simulink model "nb_spect_r2"  (R2012b)
settings: Solver=ode45  StartTime=0.0  StopTime=50000  RelTol=1e-3
undefined symbols (not defined in the file): pfb_coeff_gen_calc, sigbuilder_block, xlipgetpartsetting
libraries: xbsIndex_r4 x12159, casper_library_misc x81, casper_library_delays x40, simulink x17, dspsigops x12, xps_library x8, xbsReplacements_r4 x4, casper_library_flow_control x2
(part 6 of 142)

== system nb_spect_r2/packetizer ==
  din_valid : Inport
  din : Inport  Port=2
  reset : Inport  Port=3
  Counter : xbsIndex_r4/Counter  cnt_type=Free Running  cnt_to=Inf  operation=Up  start_count=0  cnt_by_val=1  arith_type=Unsigned  n_bits=11  bin_pt=0  load_pin=off  rst=on  en=on  explicit_period=on  period=1  dbl_ovrd=off  use_behavioral_HDL=off  implementation=Fabric  use_rpm=off  block_type=counter
  Inverter : xbsIndex_r4/Inverter  en=off  latency=0  dbl_ovrd=off  block_type=inv
  Logical : xbsIndex_r4/Logical  logical_function=AND  inputs=2  en=off  latency=0  precision=Full  arith_type=Unsigned  n_bits=16  bin_pt=0  align_bp=on  dbl_ovrd=off  block_type=logical
  Logical1 : xbsIndex_r4/Logical  logical_function=AND  inputs=2  en=off  latency=0  precision=Full  arith_type=Unsigned  n_bits=16  bin_pt=0  align_bp=on  dbl_ovrd=off  block_type=logical
  control_fsm : xbsIndex_r4/MCode  mfname=packetizer_fsm  explicit_period=on  period=1  inputsTable={'boundInpExpr'=>['','','3','',' 2047 ',''],'inputs'=>['fifo_empty','shift_count','data_per_word','data_count','n_words','reset']}  outputsTable={'outputs'=>['fifo_re','bram_addr_en','bram_we','serializer_shift','serializer_ld','shift_count_en','shift_count_rst','bram_addr_rst','data_count_en','data_count_rst','done'],'suppressOut'=>['off','off','off','off','off','off','off','off','off','off','off']}  dbl_ovrd=off  enable_stdout=off  enable_debug=off  suppress_output=1  defparams={'data_per_word',1, 'n_words', 8191 }  hide_port_list={}  block_type=mcode
      settings: block_version=10.1.3
  data_buffer : xbsIndex_r4/FIFO  mem_type=Block RAM  performance_options=Standard_FIFO  infoedit1=Available only for V4, V5, V6, V7, K7, A7 and Zynq devices.  embedded_registers=off  depth=4K  percent_nbits=8  rst=on  en=off  use_dcount=off  use_percent_full_port=on  use_almost_empty=off  almost_empty_thresh=2  use_almost_full=off  almost_full_thresh=14  dbl_ovrd=off  explicit_period=off  block_type=fifo
      settings: block_version=10.1.3
  data_counter : xbsIndex_r4/Counter  cnt_type=Free Running  cnt_to=Inf  operation=Up  start_count=0  cnt_by_val=1  arith_type=Unsigned  n_bits=14  bin_pt=0  load_pin=off  rst=on  en=on  explicit_period=on  period=1  dbl_ovrd=off  use_behavioral_HDL=off  implementation=Fabric  use_rpm=off  block_type=counter
  parallel_to_serial_converter : Subsystem  AncestorBlock=casper_library_flow_control/parallel_to_serial_converter  mask(parallel_to_serial_converter){pin_width=128, sout_width=64}
      mask prompts: pin_width "Parallel Input Width"; sout_width "Serial Output Width"
      mask help:
      | This block takes as input a parallel bus of specified width.
      | When the load signal 'ld' is asserted, this data is broken into
      | pieces of width specified by the serial output width and
      | stored into different registers chained to form a shift register.
      | If the 'shift' input is subsequently asserted, the shift register
      | returns as output a new piece of data of width sout_width.  This data
      | is the next least significant piece of the original bus.  The converter
      | serializes SMALL ENDIAN.
      |
      | Note that the load operation automatically loads the least significant
      | bits into the register closest to the output, so the first 'shift'
      | assertion changes the data output from bits [sout_width-1:0] to
      | bits [2*sout_width-1:sout_width].
      mask init:
      | parallel_to_serial_converter_init(gcb, ...
      |     'pin_width', pin_width, ...
      |     'sout_width', sout_width);
  shift_counter : xbsIndex_r4/Counter  cnt_type=Free Running  cnt_to=Inf  operation=Up  start_count=0  cnt_by_val=1  arith_type=Unsigned  n_bits=1  bin_pt=0  load_pin=off  rst=on  en=on  explicit_period=on  period=1  dbl_ovrd=off  use_behavioral_HDL=off  implementation=Fabric  use_rpm=off  block_type=counter
  data_addr : Outport
  data_sout : Outport  Port=2
  data_valid : Outport  Port=3
  buffer_overflow : Outport  Port=4
  perc_full : Outport  Port=5
  done : Outport  Port=6
  wires:
  control_fsm/10 -> data_counter/1
  reset/1 -> data_buffer/4, control_fsm/4
  data_counter/1 -> control_fsm/3
  control_fsm/9 -> data_counter/2
  control_fsm/8 -> Counter/1
  control_fsm/2 -> Counter/2
  Counter/1 -> data_addr/1
  data_buffer/2 -> control_fsm/1
  control_fsm/7 -> shift_counter/1
  shift_counter/1 -> control_fsm/2
  control_fsm/6 -> shift_counter/2
  parallel_to_serial_converter/1(sout) -> data_sout/1
  din/1 -> data_buffer/1
  control_fsm/3 -> data_valid/1
  control_fsm/5 -> parallel_to_serial_converter/2(ld)
  control_fsm/4 -> parallel_to_serial_converter/3(shift)
  control_fsm/1 -> data_buffer/3
  data_buffer/1 -> parallel_to_serial_converter/1(pin)
  Logical/1 -> data_buffer/2
  din_valid/1 -> Logical/1, Logical1/1
  Inverter/1 -> Logical/2
  data_buffer/4 -> Inverter/1, Logical1/2
  Logical1/1 -> buffer_overflow/1
  data_buffer/3 -> perc_full/1
  control_fsm/11 -> done/1

== system nb_spect_r2/pfb_fir_async ==
  sync : Inport
  dv : Inport  Port=2
  pol1_in1 : Inport  Port=3
  dv_delay : xbsIndex_r4/Delay  rst=off  infoeditControl=Selection of Reset will increase slice count due to use of real FFs and instead of SRLs  en=off  latency=bram_latency+1  dbl_ovrd=off  reg_retiming=off  block_type=delay
      settings: block_version=11.4
  pol1_in1_coeffs : Subsystem  AncestorBlock=casper_library_pfbs/pfb_coeff_gen  mask(pfb_coeff_gen){PFBSize=12, CoeffBitWidth=8, TotalTaps=6, CoeffDistMem=off, WindowType=hann, bram_latency=3, n_inputs=0, nput=0, fwidth=1, debug_mode=off, fan_latency=3}
      mask prompts: PFBSize "Size of PFB: (2^? pnts)"; CoeffBitWidth "Bitwidth of Coefficients:"; TotalTaps "Total Number of Taps:"; CoeffDistMem "Implement Coeff Gen in Distributed Memory"; WindowType "Windowing Function:"; bram_latency "BRAM Latency"; n_inputs "Number of Simultaneous Inputs: (2^?)"; nput "This is input number:"; fwidth "Bin Width (normal=1)"; debug_mode "Debug mode - coeffs are a [1:pfb_size*taps] ramp."; fan_latency "Fanout latency"
      mask init:
      | pfb_coeff_gen_init(gcb, ...
      |     'PFBSize', PFBSize, ...
      |     'CoeffBitWidth', CoeffBitWidth, ...
      |     'TotalTaps', TotalTaps, ...
      |     'CoeffDistMem', CoeffDistMem, ...
      |     'WindowType', WindowType, ...
      |     'bram_latency', bram_latency, ...
      |     'n_inputs', n_inputs, ...
      |     'nput', nput, ...
      |     'fwidth', fwidth, ...
      |     'fan_latency', fan_latency, ...
      |     'debug_mode', debug_mode);
      settings: AttributesFormatString=|
      | PFBSize=12, n_inputs=0,
      | taps=6, input=0
  pol1_in1_last_tap : Subsystem  AncestorBlock=casper_library_pfbs/last_tap_async  mask(last_tap_async){input_num=1, total_taps=6, data_in_bits=18, data_out_bits=18, coeff_bits=8, add_latency=3, mult_latency=5, quantization=Round  (unbiased: Even Values), use_hdl=on, use_embedded=off, async=on, debug_mode=off}
      mask prompts: input_num "Input number:"; total_taps "Total Number of Taps:"; data_in_bits "Input Bitwidth:"; data_out_bits "Output Bitwidth:"; coeff_bits "Coeff Bitwidth:"; add_latency "Add Latency"; mult_latency "Mult Latency"; quantization "Quantization Behavior"; use_hdl "Use behavioral HDL for multlipliers"; use_embedded "Use embedded multipliers"; async "Make asynchronous?"; debug_mode "Debug mode - coeffs are a [1:pfb_size*taps] ramp."
      mask init:
      | last_tap_async_init(gcb,...
      |     'input_num', input_num, ...
      |     'total_taps', total_taps,...
      |     'data_in_bits', data_in_bits,...
      |     'data_out_bits', data_out_bits,...
      |     'coeff_bits', coeff_bits,...
      |     'add_latency', add_latency,...
      |     'mult_latency', mult_latency,...
      |     'quantization', quantization,...
      |     'use_hdl', use_hdl,...
      |     'use_embedded', use_embedded, ...
      |     'async', async, ...
      |     'debug_mode', debug_mode);
      settings: AttributesFormatString=input(1), tap(6,6)
      mask TypeOptions quantization: Truncate | Round  (unbiased: +/- Inf) | Round  (unbiased: Even Values)
      mask Callback use_hdl:
      | use_hdl = get_param(gcb,'use_hdl');
      | if( strcmp(use_hdl,'on')),
      |     set_param(gcb, 'use_embedded','off');
      |     set_param(gcb, 'MaskVisibilities',{'on','on','on','on','on','on','on','on','on','off', 'on', 'on'});
      | else
      |     set_param(gcb, 'MaskVisibilities',{'on','on','on','on','on','on','on','on','on','on', 'on', 'on'});
      | end
  pol1_in1_tap1 : Subsystem  AncestorBlock=casper_library_pfbs/tap_async  mask(tap_async){this_tap=1, pfb_bits=12, coeff_bits=8, total_taps=6, data_in_bits=18, mult_latency=5, bram_latency=3, simul_bits=0, fwidth=1, use_hdl=on, use_embedded=off, async=on, debug_mode=off}
      mask prompts: this_tap "Tap number:"; pfb_bits "Size of PFB: (2^? pnts)"; coeff_bits "Bitwidth of Coefficients:"; total_taps "Total Number of Taps:"; data_in_bits "Input Bitwidth:"; mult_latency "Mult Latency"; bram_latency "BRAM Latency"; simul_bits "Number of Simultaneous Inputs: (2^?)"; fwidth "Bit Width (normal=1)"; use_hdl "Use behavioral HDL for multlipliers"; use_embedded "Use embedded multipliers"; async "Make asynchronous?"; debug_mode "Debug mode - coeffs are a [1:pfb_size*taps] ramp."
      mask init:
      | pfb_async_tap_init(gcb,...
      |     'this_tap', this_tap, ...
      |     'pfb_bits', pfb_bits,...
      |     'coeff_bits', coeff_bits,...
      |     'total_taps', total_taps,...
      |     'data_in_bits', data_in_bits,...
      |     'mult_latency', mult_latency,...
      |     'bram_latency', bram_latency,...
      |     'simul_bits', simul_bits,...
      |     'fwidth', fwidth,...
      |     'use_hdl', use_hdl,...
      |     'use_embedded', use_embedded,...
      |     'async', async, ...
      |     'debug_mode', debug_mode);
      settings: AttributesFormatString=tap(1/6)
      mask Callback use_hdl:
      | use_hdl = get_param(gcb,'use_hdl');
      | if( strcmp(use_hdl,'on')),
      |     set_param(gcb, 'use_embedded','off');
      |     set_param(gcb, 'MaskVisibilities',{'on','on','on','on','on','on','on','on','on','on','off','on', 'on'});
      | else,
      |     set_param(gcb, 'MaskVisibilities',{'on','on','on','on','on','on','on','on','on','on','on','on', 'on'});
      | end
  pol1_in1_tap2 : Subsystem  AncestorBlock=casper_library_pfbs/tap_async  mask(tap_async){this_tap=2, pfb_bits=12, coeff_bits=8, total_taps=6, data_in_bits=18, mult_latency=5, bram_latency=3, simul_bits=0, fwidth=1, use_hdl=on, use_embedded=off, async=on, debug_mode=off}
      mask prompts: this_tap "Tap number:"; pfb_bits "Size of PFB: (2^? pnts)"; coeff_bits "Bitwidth of Coefficients:"; total_taps "Total Number of Taps:"; data_in_bits "Input Bitwidth:"; mult_latency "Mult Latency"; bram_latency "BRAM Latency"; simul_bits "Number of Simultaneous Inputs: (2^?)"; fwidth "Bit Width (normal=1)"; use_hdl "Use behavioral HDL for multlipliers"; use_embedded "Use embedded multipliers"; async "Make asynchronous?"; debug_mode "Debug mode - coeffs are a [1:pfb_size*taps] ramp."
      mask init: same as nb_spect_r2/pfb_fir_async/pol1_in1_tap1
      settings: AttributesFormatString=tap(2/6)
      mask Callback use_hdl:
      | use_hdl = get_param(gcb,'use_hdl');
      | if( strcmp(use_hdl,'on')),
      |     set_param(gcb, 'use_embedded','off');
      |     set_param(gcb, 'MaskVisibilities',{'on','on','on','on','on','on','on','on','on','on','off','on', 'on'});
      | else,
      |     set_param(gcb, 'MaskVisibilities',{'on','on','on','on','on','on','on','on','on','on','on','on', 'on'});
      | end
  pol1_in1_tap3 : Subsystem  AncestorBlock=casper_library_pfbs/tap_async  mask(tap_async){this_tap=3, pfb_bits=12, coeff_bits=8, total_taps=6, data_in_bits=18, mult_latency=5, bram_latency=3, simul_bits=0, fwidth=1, use_hdl=on, use_embedded=off, async=on, debug_mode=off}
      mask prompts: this_tap "Tap number:"; pfb_bits "Size of PFB: (2^? pnts)"; coeff_bits "Bitwidth of Coefficients:"; total_taps "Total Number of Taps:"; data_in_bits "Input Bitwidth:"; mult_latency "Mult Latency"; bram_latency "BRAM Latency"; simul_bits "Number of Simultaneous Inputs: (2^?)"; fwidth "Bit Width (normal=1)"; use_hdl "Use behavioral HDL for multlipliers"; use_embedded "Use embedded multipliers"; async "Make asynchronous?"; debug_mode "Debug mode - coeffs are a [1:pfb_size*taps] ramp."
      mask init: same as nb_spect_r2/pfb_fir_async/pol1_in1_tap1
      settings: AttributesFormatString=tap(3/6)
      mask Callback use_hdl:
      | use_hdl = get_param(gcb,'use_hdl');
      | if( strcmp(use_hdl,'on')),
      |     set_param(gcb, 'use_embedded','off');
      |     set_param(gcb, 'MaskVisibilities',{'on','on','on','on','on','on','on','on','on','on','off','on', 'on'});
      | else,
      |     set_param(gcb, 'MaskVisibilities',{'on','on','on','on','on','on','on','on','on','on','on','on', 'on'});
      | end
  pol1_in1_tap4 : Subsystem  AncestorBlock=casper_library_pfbs/tap_async  mask(tap_async){this_tap=4, pfb_bits=12, coeff_bits=8, total_taps=6, data_in_bits=18, mult_latency=5, bram_latency=3, simul_bits=0, fwidth=1, use_hdl=on, use_embedded=off, async=on, debug_mode=off}
      mask prompts: this_tap "Tap number:"; pfb_bits "Size of PFB: (2^? pnts)"; coeff_bits "Bitwidth of Coefficients:"; total_taps "Total Number of Taps:"; data_in_bits "Input Bitwidth:"; mult_latency "Mult Latency"; bram_latency "BRAM Latency"; simul_bits "Number of Simultaneous Inputs: (2^?)"; fwidth "Bit Width (normal=1)"; use_hdl "Use behavioral HDL for multlipliers"; use_embedded "Use embedded multipliers"; async "Make asynchronous?"; debug_mode "Debug mode - coeffs are a [1:pfb_size*taps] ramp."
      mask init: same as nb_spect_r2/pfb_fir_async/pol1_in1_tap1
      settings: AttributesFormatString=tap(4/6)
      mask Callback use_hdl:
      | use_hdl = get_param(gcb,'use_hdl');
      | if( strcmp(use_hdl,'on')),
      |     set_param(gcb, 'use_embedded','off');
      |     set_param(gcb, 'MaskVisibilities',{'on','on','on','on','on','on','on','on','on','on','off','on', 'on'});
      | else,
      |     set_param(gcb, 'MaskVisibilities',{'on','on','on','on','on','on','on','on','on','on','on','on', 'on'});
      | end
  pol1_in1_tap5 : Subsystem  AncestorBlock=casper_library_pfbs/tap_async  mask(tap_async){this_tap=5, pfb_bits=12, coeff_bits=8, total_taps=6, data_in_bits=18, mult_latency=5, bram_latency=3, simul_bits=0, fwidth=1, use_hdl=on, use_embedded=off, async=on, debug_mode=off}
      mask prompts: this_tap "Tap number:"; pfb_bits "Size of PFB: (2^? pnts)"; coeff_bits "Bitwidth of Coefficients:"; total_taps "Total Number of Taps:"; data_in_bits "Input Bitwidth:"; mult_latency "Mult Latency"; bram_latency "BRAM Latency"; simul_bits "Number of Simultaneous Inputs: (2^?)"; fwidth "Bit Width (normal=1)"; use_hdl "Use behavioral HDL for multlipliers"; use_embedded "Use embedded multipliers"; async "Make asynchronous?"; debug_mode "Debug mode - coeffs are a [1:pfb_size*taps] ramp."
      mask init: same as nb_spect_r2/pfb_fir_async/pol1_in1_tap1
      settings: AttributesFormatString=tap(5/6)
      mask Callback use_hdl:
      | use_hdl = get_param(gcb,'use_hdl');
      | if( strcmp(use_hdl,'on')),
      |     set_param(gcb, 'use_embedded','off');
      |     set_param(gcb, 'MaskVisibilities',{'on','on','on','on','on','on','on','on','on','on','off','on', 'on'});
      | else,
      |     set_param(gcb, 'MaskVisibilities',{'on','on','on','on','on','on','on','on','on','on','on','on', 'on'});
      | end
  sync_generate : Subsystem
  sync_out : Outport
  dv_out : Outport  Port=2
  pol1_out1 : Outport  Port=3
  wires:
  dv/1 -> dv_delay/1
  pol1_in1/1 -> pol1_in1_coeffs/1(din)
  sync/1 -> pol1_in1_coeffs/2(sync)
  pol1_in1_coeffs/1(dout) -> pol1_in1_tap1/1(din)
  pol1_in1_coeffs/2(sync_out) -> pol1_in1_tap1/2(sync), sync_generate/1(sync)
  pol1_in1_coeffs/3(coeff) -> pol1_in1_tap1/3(coeffs)
  dv_delay/1 -> pol1_in1_tap1/4(dvin), sync_generate/2(dv)
  pol1_in1_tap1/1(dout) -> pol1_in1_tap2/1(din)
  pol1_in1_tap1/2(sync_out) -> pol1_in1_tap2/2(sync)
  pol1_in1_tap1/3(coeff_out) -> pol1_in1_tap2/3(coeffs)
  pol1_in1_tap1/4(dv_out) -> pol1_in1_tap2/4(dvin)
  pol1_in1_tap1/5(taps_out) -> pol1_in1_tap2/5(taps_in)
  pol1_in1_tap2/1(dout) -> pol1_in1_tap3/1(din)
  pol1_in1_tap2/2(sync_out) -> pol1_in1_tap3/2(sync)
  pol1_in1_tap2/3(coeff_out) -> pol1_in1_tap3/3(coeffs)
  pol1_in1_tap2/4(dv_out) -> pol1_in1_tap3/4(dvin)
  pol1_in1_tap2/5(taps_out) -> pol1_in1_tap3/5(taps_in)
  pol1_in1_tap3/1(dout) -> pol1_in1_tap4/1(din)
  pol1_in1_tap3/2(sync_out) -> pol1_in1_tap4/2(sync)
  pol1_in1_tap3/3(coeff_out) -> pol1_in1_tap4/3(coeffs)
  pol1_in1_tap3/4(dv_out) -> pol1_in1_tap4/4(dvin)
  pol1_in1_tap3/5(taps_out) -> pol1_in1_tap4/5(taps_in)
  pol1_in1_tap4/1(dout) -> pol1_in1_tap5/1(din)
  pol1_in1_tap4/2(sync_out) -> pol1_in1_tap5/2(sync)
  pol1_in1_tap4/3(coeff_out) -> pol1_in1_tap5/3(coeffs)
  pol1_in1_tap4/4(dv_out) -> pol1_in1_tap5/4(dvin)
  pol1_in1_tap4/5(taps_out) -> pol1_in1_tap5/5(taps_in)
  pol1_in1_last_tap/1(dout) -> pol1_out1/1
  pol1_in1_last_tap/2(sync_out) -> sync_out/1
  pol1_in1_last_tap/3(dv_out) -> dv_out/1
  pol1_in1_tap5/1(dout) -> pol1_in1_last_tap/1(din)
  pol1_in1_tap5/3(coeff_out) -> pol1_in1_last_tap/3(coeff)
  pol1_in1_tap5/4(dv_out) -> pol1_in1_last_tap/4(dvin)
  pol1_in1_tap5/5(taps_out) -> pol1_in1_last_tap/5(taps_in)
  sync_generate/1(sync_out) -> pol1_in1_last_tap/2(sync)

== system nb_spect_r2/pfb_fir_async1 ==
  sync : Inport
  dv : Inport  Port=2
  pol1_in1 : Inport  Port=3
  dv_delay : xbsIndex_r4/Delay  rst=off  infoeditControl=Selection of Reset will increase slice count due to use of real FFs and instead of SRLs  en=off  latency=bram_latency+1  dbl_ovrd=off  reg_retiming=off  block_type=delay
      settings: block_version=11.4
  pol1_in1_coeffs : Subsystem  AncestorBlock=casper_library_pfbs/pfb_coeff_gen  mask(pfb_coeff_gen){PFBSize=12, CoeffBitWidth=8, TotalTaps=6, CoeffDistMem=off, WindowType=hann, bram_latency=3, n_inputs=0, nput=0, fwidth=1, debug_mode=off, fan_latency=3}
      mask prompts: PFBSize "Size of PFB: (2^? pnts)"; CoeffBitWidth "Bitwidth of Coefficients:"; TotalTaps "Total Number of Taps:"; CoeffDistMem "Implement Coeff Gen in Distributed Memory"; WindowType "Windowing Function:"; bram_latency "BRAM Latency"; n_inputs "Number of Simultaneous Inputs: (2^?)"; nput "This is input number:"; fwidth "Bin Width (normal=1)"; debug_mode "Debug mode - coeffs are a [1:pfb_size*taps] ramp."; fan_latency "Fanout latency"
      mask init: same as nb_spect_r2/pfb_fir_async/pol1_in1_coeffs
      settings: AttributesFormatString=|
      | PFBSize=12, n_inputs=0,
      | taps=6, input=0
  pol1_in1_last_tap : Subsystem  AncestorBlock=casper_library_pfbs/last_tap_async  mask(last_tap_async){input_num=1, total_taps=6, data_in_bits=18, data_out_bits=18, coeff_bits=8, add_latency=3, mult_latency=5, quantization=Round  (unbiased: Even Values), use_hdl=on, use_embedded=off, async=on, debug_mode=off}
      mask prompts: input_num "Input number:"; total_taps "Total Number of Taps:"; data_in_bits "Input Bitwidth:"; data_out_bits "Output Bitwidth:"; coeff_bits "Coeff Bitwidth:"; add_latency "Add Latency"; mult_latency "Mult Latency"; quantization "Quantization Behavior"; use_hdl "Use behavioral HDL for multlipliers"; use_embedded "Use embedded multipliers"; async "Make asynchronous?"; debug_mode "Debug mode - coeffs are a [1:pfb_size*taps] ramp."
      mask init: same as nb_spect_r2/pfb_fir_async/pol1_in1_last_tap
      settings: AttributesFormatString=input(1), tap(6,6)
      mask TypeOptions quantization: Truncate | Round  (unbiased: +/- Inf) | Round  (unbiased: Even Values)
      mask Callback use_hdl:
      | use_hdl = get_param(gcb,'use_hdl');
      | if( strcmp(use_hdl,'on')),
      |     set_param(gcb, 'use_embedded','off');
      |     set_param(gcb, 'MaskVisibilities',{'on','on','on','on','on','on','on','on','on','off', 'on', 'on'});
      | else
      |     set_param(gcb, 'MaskVisibilities',{'on','on','on','on','on','on','on','on','on','on', 'on', 'on'});
      | end
  pol1_in1_tap1 : Subsystem  AncestorBlock=casper_library_pfbs/tap_async  mask(tap_async){this_tap=1, pfb_bits=12, coeff_bits=8, total_taps=6, data_in_bits=18, mult_latency=5, bram_latency=3, simul_bits=0, fwidth=1, use_hdl=on, use_embedded=off, async=on, debug_mode=off}
      mask prompts: this_tap "Tap number:"; pfb_bits "Size of PFB: (2^? pnts)"; coeff_bits "Bitwidth of Coefficients:"; total_taps "Total Number of Taps:"; data_in_bits "Input Bitwidth:"; mult_latency "Mult Latency"; bram_latency "BRAM Latency"; simul_bits "Number of Simultaneous Inputs: (2^?)"; fwidth "Bit Width (normal=1)"; use_hdl "Use behavioral HDL for multlipliers"; use_embedded "Use embedded multipliers"; async "Make asynchronous?"; debug_mode "Debug mode - coeffs are a [1:pfb_size*taps] ramp."
      mask init: same as nb_spect_r2/pfb_fir_async/pol1_in1_tap1
      settings: AttributesFormatString=tap(1/6)
      mask Callback use_hdl:
      | use_hdl = get_param(gcb,'use_hdl');
      | if( strcmp(use_hdl,'on')),
      |     set_param(gcb, 'use_embedded','off');
      |     set_param(gcb, 'MaskVisibilities',{'on','on','on','on','on','on','on','on','on','on','off','on', 'on'});
      | else,
      |     set_param(gcb, 'MaskVisibilities',{'on','on','on','on','on','on','on','on','on','on','on','on', 'on'});
      | end
  pol1_in1_tap2 : Subsystem  AncestorBlock=casper_library_pfbs/tap_async  mask(tap_async){this_tap=2, pfb_bits=12, coeff_bits=8, total_taps=6, data_in_bits=18, mult_latency=5, bram_latency=3, simul_bits=0, fwidth=1, use_hdl=on, use_embedded=off, async=on, debug_mode=off}
      mask prompts: this_tap "Tap number:"; pfb_bits "Size of PFB: (2^? pnts)"; coeff_bits "Bitwidth of Coefficients:"; total_taps "Total Number of Taps:"; data_in_bits "Input Bitwidth:"; mult_latency "Mult Latency"; bram_latency "BRAM Latency"; simul_bits "Number of Simultaneous Inputs: (2^?)"; fwidth "Bit Width (normal=1)"; use_hdl "Use behavioral HDL for multlipliers"; use_embedded "Use embedded multipliers"; async "Make asynchronous?"; debug_mode "Debug mode - coeffs are a [1:pfb_size*taps] ramp."
      mask init: same as nb_spect_r2/pfb_fir_async/pol1_in1_tap1
      settings: AttributesFormatString=tap(2/6)
      mask Callback use_hdl:
      | use_hdl = get_param(gcb,'use_hdl');
      | if( strcmp(use_hdl,'on')),
      |     set_param(gcb, 'use_embedded','off');
      |     set_param(gcb, 'MaskVisibilities',{'on','on','on','on','on','on','on','on','on','on','off','on', 'on'});
      | else,
      |     set_param(gcb, 'MaskVisibilities',{'on','on','on','on','on','on','on','on','on','on','on','on', 'on'});
      | end
  pol1_in1_tap3 : Subsystem  AncestorBlock=casper_library_pfbs/tap_async  mask(tap_async){this_tap=3, pfb_bits=12, coeff_bits=8, total_taps=6, data_in_bits=18, mult_latency=5, bram_latency=3, simul_bits=0, fwidth=1, use_hdl=on, use_embedded=off, async=on, debug_mode=off}
      mask prompts: this_tap "Tap number:"; pfb_bits "Size of PFB: (2^? pnts)"; coeff_bits "Bitwidth of Coefficients:"; total_taps "Total Number of Taps:"; data_in_bits "Input Bitwidth:"; mult_latency "Mult Latency"; bram_latency "BRAM Latency"; simul_bits "Number of Simultaneous Inputs: (2^?)"; fwidth "Bit Width (normal=1)"; use_hdl "Use behavioral HDL for multlipliers"; use_embedded "Use embedded multipliers"; async "Make asynchronous?"; debug_mode "Debug mode - coeffs are a [1:pfb_size*taps] ramp."
      mask init: same as nb_spect_r2/pfb_fir_async/pol1_in1_tap1
      settings: AttributesFormatString=tap(3/6)
      mask Callback use_hdl:
      | use_hdl = get_param(gcb,'use_hdl');
      | if( strcmp(use_hdl,'on')),
      |     set_param(gcb, 'use_embedded','off');
      |     set_param(gcb, 'MaskVisibilities',{'on','on','on','on','on','on','on','on','on','on','off','on', 'on'});
      | else,
      |     set_param(gcb, 'MaskVisibilities',{'on','on','on','on','on','on','on','on','on','on','on','on', 'on'});
      | end
  pol1_in1_tap4 : Subsystem  AncestorBlock=casper_library_pfbs/tap_async  mask(tap_async){this_tap=4, pfb_bits=12, coeff_bits=8, total_taps=6, data_in_bits=18, mult_latency=5, bram_latency=3, simul_bits=0, fwidth=1, use_hdl=on, use_embedded=off, async=on, debug_mode=off}
      mask prompts: this_tap "Tap number:"; pfb_bits "Size of PFB: (2^? pnts)"; coeff_bits "Bitwidth of Coefficients:"; total_taps "Total Number of Taps:"; data_in_bits "Input Bitwidth:"; mult_latency "Mult Latency"; bram_latency "BRAM Latency"; simul_bits "Number of Simultaneous Inputs: (2^?)"; fwidth "Bit Width (normal=1)"; use_hdl "Use behavioral HDL for multlipliers"; use_embedded "Use embedded multipliers"; async "Make asynchronous?"; debug_mode "Debug mode - coeffs are a [1:pfb_size*taps] ramp."
      mask init: same as nb_spect_r2/pfb_fir_async/pol1_in1_tap1
      settings: AttributesFormatString=tap(4/6)
      mask Callback use_hdl:
      | use_hdl = get_param(gcb,'use_hdl');
      | if( strcmp(use_hdl,'on')),
      |     set_param(gcb, 'use_embedded','off');
      |     set_param(gcb, 'MaskVisibilities',{'on','on','on','on','on','on','on','on','on','on','off','on', 'on'});
      | else,
      |     set_param(gcb, 'MaskVisibilities',{'on','on','on','on','on','on','on','on','on','on','on','on', 'on'});
      | end
  pol1_in1_tap5 : Subsystem  AncestorBlock=casper_library_pfbs/tap_async  mask(tap_async){this_tap=5, pfb_bits=12, coeff_bits=8, total_taps=6, data_in_bits=18, mult_latency=5, bram_latency=3, simul_bits=0, fwidth=1, use_hdl=on, use_embedded=off, async=on, debug_mode=off}
      mask prompts: this_tap "Tap number:"; pfb_bits "Size of PFB: (2^? pnts)"; coeff_bits "Bitwidth of Coefficients:"; total_taps "Total Number of Taps:"; data_in_bits "Input Bitwidth:"; mult_latency "Mult Latency"; bram_latency "BRAM Latency"; simul_bits "Number of Simultaneous Inputs: (2^?)"; fwidth "Bit Width (normal=1)"; use_hdl "Use behavioral HDL for multlipliers"; use_embedded "Use embedded multipliers"; async "Make asynchronous?"; debug_mode "Debug mode - coeffs are a [1:pfb_size*taps] ramp."
      mask init: same as nb_spect_r2/pfb_fir_async/pol1_in1_tap1
      settings: AttributesFormatString=tap(5/6)
      mask Callback use_hdl:
      | use_hdl = get_param(gcb,'use_hdl');
      | if( strcmp(use_hdl,'on')),
      |     set_param(gcb, 'use_embedded','off');
      |     set_param(gcb, 'MaskVisibilities',{'on','on','on','on','on','on','on','on','on','on','off','on', 'on'});
      | else,
      |     set_param(gcb, 'MaskVisibilities',{'on','on','on','on','on','on','on','on','on','on','on','on', 'on'});
      | end
  sync_generate : Subsystem
  sync_out : Outport
  dv_out : Outport  Port=2
  pol1_out1 : Outport  Port=3
  wires:
  dv/1 -> dv_delay/1
  pol1_in1/1 -> pol1_in1_coeffs/1(din)
  sync/1 -> pol1_in1_coeffs/2(sync)
  pol1_in1_coeffs/1(dout) -> pol1_in1_tap1/1(din)
  pol1_in1_coeffs/2(sync_out) -> pol1_in1_tap1/2(sync), sync_generate/1(sync)
  pol1_in1_coeffs/3(coeff) -> pol1_in1_tap1/3(coeffs)
  dv_delay/1 -> pol1_in1_tap1/4(dvin), sync_generate/2(dv)
  pol1_in1_tap1/1(dout) -> pol1_in1_tap2/1(din)
  pol1_in1_tap1/2(sync_out) -> pol1_in1_tap2/2(sync)
  pol1_in1_tap1/3(coeff_out) -> pol1_in1_tap2/3(coeffs)
  pol1_in1_tap1/4(dv_out) -> pol1_in1_tap2/4(dvin)
  pol1_in1_tap1/5(taps_out) -> pol1_in1_tap2/5(taps_in)
  pol1_in1_tap2/1(dout) -> pol1_in1_tap3/1(din)
  pol1_in1_tap2/2(sync_out) -> pol1_in1_tap3/2(sync)
  pol1_in1_tap2/3(coeff_out) -> pol1_in1_tap3/3(coeffs)
  pol1_in1_tap2/4(dv_out) -> pol1_in1_tap3/4(dvin)
  pol1_in1_tap2/5(taps_out) -> pol1_in1_tap3/5(taps_in)
  pol1_in1_tap3/1(dout) -> pol1_in1_tap4/1(din)
  pol1_in1_tap3/2(sync_out) -> pol1_in1_tap4/2(sync)
  pol1_in1_tap3/3(coeff_out) -> pol1_in1_tap4/3(coeffs)
  pol1_in1_tap3/4(dv_out) -> pol1_in1_tap4/4(dvin)
  pol1_in1_tap3/5(taps_out) -> pol1_in1_tap4/5(taps_in)
  pol1_in1_tap4/1(dout) -> pol1_in1_tap5/1(din)
  pol1_in1_tap4/2(sync_out) -> pol1_in1_tap5/2(sync)
  pol1_in1_tap4/3(coeff_out) -> pol1_in1_tap5/3(coeffs)
  pol1_in1_tap4/4(dv_out) -> pol1_in1_tap5/4(dvin)
  pol1_in1_tap4/5(taps_out) -> pol1_in1_tap5/5(taps_in)
  pol1_in1_last_tap/1(dout) -> pol1_out1/1
  pol1_in1_last_tap/2(sync_out) -> sync_out/1
  pol1_in1_last_tap/3(dv_out) -> dv_out/1
  pol1_in1_tap5/1(dout) -> pol1_in1_last_tap/1(din)
  pol1_in1_tap5/3(coeff_out) -> pol1_in1_last_tap/3(coeff)
  pol1_in1_tap5/4(dv_out) -> pol1_in1_last_tap/4(dvin)
  pol1_in1_tap5/5(taps_out) -> pol1_in1_last_tap/5(taps_in)
  sync_generate/1(sync_out) -> pol1_in1_last_tap/2(sync)
